simulink model "lucrarea4_3_sim"  (R2020b)
settings: Solver=VariableStepAuto  StartTime=0.0  StopTime=0.5  RelTol=1e-3
values from neighbouring files (symbols this model uses):
  Ad = [0.7332, -0.0528; 1, 0]    [lucrarea4_2.m]    (also in lucrarea4_3.m)
  Bd = [1; 0]    [lucrarea4_2.m]    (also in lucrarea4_3.m)
  eta = 1/(Cd*(inv(X)*Bd))    [lucrarea4_3.m]
  K = -Kopt    [lucrarea4_3.m]
  Te = 0.01    [lucrarea3_3.m]    (also in lucrarea4_2.m; lucrarea4_3.m)
undefined symbols (not defined in the file or in its folder): Cd
settings Model: Creator=student  LastModifiedBy=student

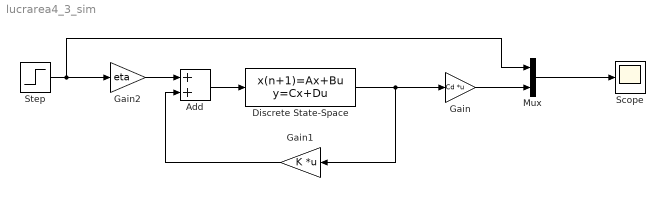
== system lucrarea4_3_sim ==
  Add : Sum
  Discrete State-Space : DiscreteStateSpace  A=Ad  B=Bd  C=eye(2)  D=[0;0]  InitialCondition=[0;0]  SampleTime=Te
  Gain : Gain  Gain=Cd  Multiplication=Matrix(K*u)
  Gain1 : Gain  Gain=K  Multiplication=Matrix(K*u)
  Gain2 : Gain  Gain=eta
  Mux : Mux  Inputs=2
  Scope : Scope
  Step : Step  Time=0  SampleTime=0
  wires:
  Discrete State-Space/1 -> Gain/1, Gain1/1
  Step/1 -> Mux/1, Gain2/1
  Gain/1 -> Mux/2
  Mux/1 -> Scope/1
  Gain2/1 -> Add/1
  Add/1 -> Discrete State-Space/1
  Gain1/1 -> Add/2
